simulink model "BlockDiagram"  (R2023a)
settings: Solver=VariableStepAuto  StartTime=0.0  StopTime=10.0  RelTol=1e-3
libraries: visionsinks x3, visionsources x2
settings Model: Creator=thaweesaktrongtirakul  LastModifiedBy=thaweesaktrongtirakul

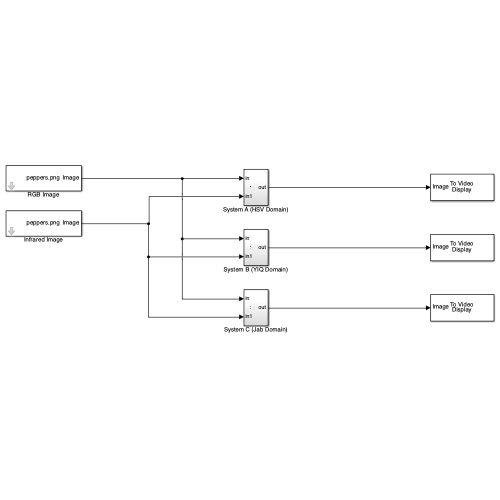
[thumbnail: Simulink's stored preview of the top-level diagram]
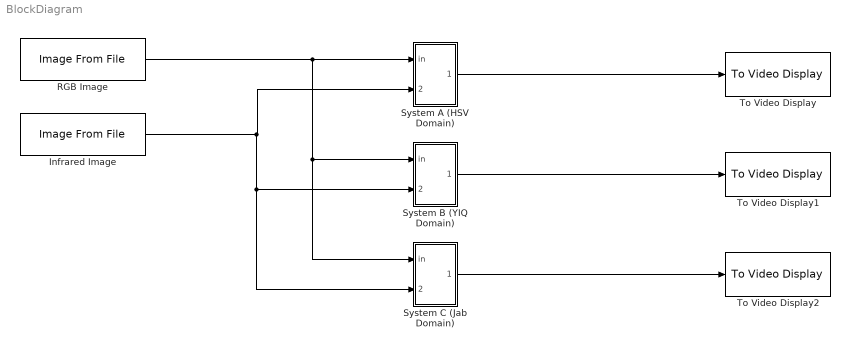
== system BlockDiagram ==
  Infrared Image : visionsources/Image From File  Tag=vipblks_nd  FileName=peppers.png  Ts=inf  imagePorts=One multidimensional signal  OutPortLabels=R|G|B  ImageDataType=Inherit from input image  sdImageDataType=uint(8)  Signed=on  WordLength=16  FractionLengthMode=User-defined  FractionLength=15
  RGB Image : visionsources/Image From File  Tag=vipblks_nd  FileName=peppers.png  Ts=inf  imagePorts=One multidimensional signal  OutPortLabels=R|G|B  ImageDataType=Inherit from input image  sdImageDataType=uint(8)  Signed=on  WordLength=16  FractionLengthMode=User-defined  FractionLength=15
  System A (HSV Domain) : Subsystem
  System B (YIQ Domain) : Subsystem
  System C (Jab Domain) : Subsystem
  To Video Display : visionsinks/To Video Display  windowSizeMode=Normal  openAtMdlStart=on  fullScreen=off  videoWindowX=536805376  videoWindowY=536805376  saveWindowSize=off  videoWindowWidth=2147483647  videoWindowHeight=2147483647  inputColorFormat=RGB  inputType=Obsolete  imagePorts=One multidimensional signal  OutputDevice=On-screen video monitor  dataOrg=Column-major  isWindowOpen=off
  To Video Display1 : visionsinks/To Video Display  windowSizeMode=Normal  openAtMdlStart=on  fullScreen=off  videoWindowX=536805376  videoWindowY=536805376  saveWindowSize=off  videoWindowWidth=2147483647  videoWindowHeight=2147483647  inputColorFormat=RGB  inputType=Obsolete  imagePorts=One multidimensional signal  OutputDevice=On-screen video monitor  dataOrg=Column-major  isWindowOpen=off
  To Video Display2 : visionsinks/To Video Display  windowSizeMode=Normal  openAtMdlStart=on  fullScreen=off  videoWindowX=536805376  videoWindowY=536805376  saveWindowSize=off  videoWindowWidth=2147483647  videoWindowHeight=2147483647  inputColorFormat=RGB  inputType=Obsolete  imagePorts=One multidimensional signal  OutputDevice=On-screen video monitor  dataOrg=Column-major  isWindowOpen=off
  wires:
  RGB Image/1 -> System C (Jab Domain)/1(in), System B (YIQ Domain)/1(in), System A (HSV Domain)/1(in)
  Infrared Image/1 -> System C (Jab Domain)/2(in1), System B (YIQ Domain)/2(in1), System A (HSV Domain)/2(in1)
  System A (HSV Domain)/1(out) -> To Video Display/1
  System B (YIQ Domain)/1(out) -> To Video Display1/1
  System C (Jab Domain)/1(out) -> To Video Display2/1

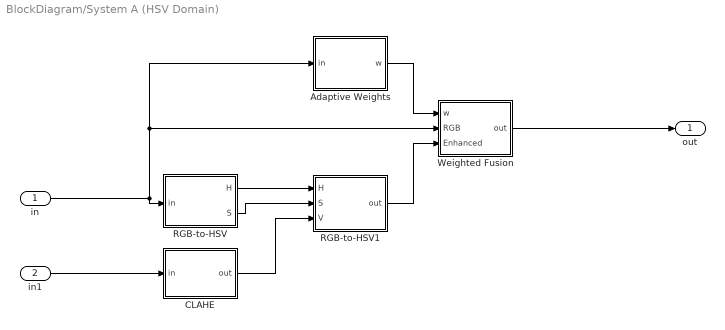
== system BlockDiagram/System A (HSV Domain) ==
  in : Inport
  in1 : Inport  Port=2
  Adaptive Weights : MATLAB Function  TreatAsAtomicUnit=on
  CLAHE : MATLAB Function  TreatAsAtomicUnit=on
  RGB-to-HSV : MATLAB Function  TreatAsAtomicUnit=on
  RGB-to-HSV1 : MATLAB Function  TreatAsAtomicUnit=on
  Weighted Fusion : MATLAB Function  TreatAsAtomicUnit=on
  out : Outport
  wires:
  Weighted Fusion/1(out) -> out/1
  in1/1 -> CLAHE/1(in)
  RGB-to-HSV1/1(out) -> Weighted Fusion/3(Enhanced)
  CLAHE/1(out) -> RGB-to-HSV1/3(V)
  RGB-to-HSV/1(H) -> RGB-to-HSV1/1(H)
  Adaptive Weights/1(w) -> Weighted Fusion/1(w)
  RGB-to-HSV/2(S) -> RGB-to-HSV1/2(S)
  in/1 -> Weighted Fusion/2(RGB), Adaptive Weights/1(in), RGB-to-HSV/1(in)

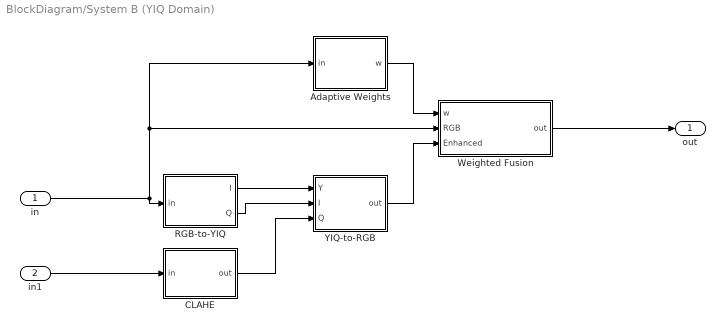
== system BlockDiagram/System B (YIQ Domain) ==
  in : Inport
  in1 : Inport  Port=2
  Adaptive Weights : MATLAB Function  TreatAsAtomicUnit=on
  CLAHE : MATLAB Function  TreatAsAtomicUnit=on
  RGB-to-YIQ : MATLAB Function  TreatAsAtomicUnit=on
  Weighted Fusion : MATLAB Function  TreatAsAtomicUnit=on
  YIQ-to-RGB : MATLAB Function  TreatAsAtomicUnit=on
  out : Outport
  wires:
  Weighted Fusion/1(out) -> out/1
  in1/1 -> CLAHE/1(in)
  YIQ-to-RGB/1(out) -> Weighted Fusion/3(Enhanced)
  CLAHE/1(out) -> YIQ-to-RGB/3(Q)
  RGB-to-YIQ/1(I) -> YIQ-to-RGB/1(Y)
  Adaptive Weights/1(w) -> Weighted Fusion/1(w)
  RGB-to-YIQ/2(Q) -> YIQ-to-RGB/2(I)
  in/1 -> Weighted Fusion/2(RGB), Adaptive Weights/1(in), RGB-to-YIQ/1(in)

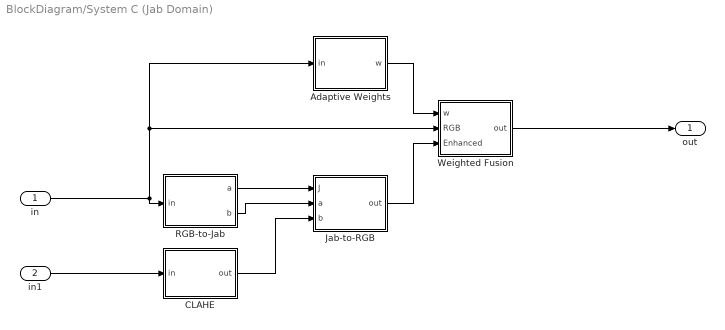
== system BlockDiagram/System C (Jab Domain) ==
  in : Inport
  in1 : Inport  Port=2
  Adaptive Weights : MATLAB Function  TreatAsAtomicUnit=on
  CLAHE : MATLAB Function  TreatAsAtomicUnit=on
  Jab-to-RGB : MATLAB Function  TreatAsAtomicUnit=on
  RGB-to-Jab : MATLAB Function  TreatAsAtomicUnit=on
  Weighted Fusion : MATLAB Function  TreatAsAtomicUnit=on
  out : Outport
  wires:
  Weighted Fusion/1(out) -> out/1
  in1/1 -> CLAHE/1(in)
  Jab-to-RGB/1(out) -> Weighted Fusion/3(Enhanced)
  CLAHE/1(out) -> Jab-to-RGB/3(b)
  RGB-to-Jab/1(a) -> Jab-to-RGB/1(J)
  Adaptive Weights/1(w) -> Weighted Fusion/1(w)
  RGB-to-Jab/2(b) -> Jab-to-RGB/2(a)
  in/1 -> Weighted Fusion/2(RGB), Adaptive Weights/1(in), RGB-to-Jab/1(in)

== matlab function BlockDiagram/System C (Jab Domain)/Weighted Fusion ==
  data: w input; RGB input; out output; Enhanced input
function out = fcn(w,RGB,Enhanced)
    out = RGB+Enhanced+w;
end

== matlab function BlockDiagram/System A (HSV Domain)/RGB-to-HSV ==
  data: in input; H output; S output
function [H,S] = fcn(in)
    H = in;
    S = in;

end

== matlab function BlockDiagram/System C (Jab Domain)/RGB-to-Jab ==
  data: in input; a output; b output
function [a,b] = fcn(in)
    a = in;
    b = in;

end

== matlab function BlockDiagram/System C (Jab Domain)/Jab-to-RGB ==
  data: J input; out output; a input; b input
function out = fcn(J,a,b)
    out = J+a+b;
end

== matlab function BlockDiagram/System A (HSV Domain)/CLAHE ==
  data: in input; out output
function out = fcn(in)
    out = in;
end

== matlab function BlockDiagram/System A (HSV Domain)/RGB-to-HSV1 ==
  data: H input; out output; S input; V input
function out = fcn(H,S,V)
    out = H+S+V;
end

== matlab function BlockDiagram/System A (HSV Domain)/Adaptive Weights ==
  data: in input; w output
function w  = fcn(in)
    w = in;
end

== matlab function BlockDiagram/System A (HSV Domain)/Weighted Fusion ==
  data: w input; RGB input; out output; Enhanced input
function out = fcn(w,RGB,Enhanced)
    out = RGB+Enhanced+w;
end

== matlab function BlockDiagram/System B (YIQ Domain)/Adaptive Weights ==
  data: in input; w output
function w  = fcn(in)
    w = in;
end

== matlab function BlockDiagram/System B (YIQ Domain)/CLAHE ==
  data: in input; out output
function out = fcn(in)
    out = in;
end

== matlab function BlockDiagram/System B (YIQ Domain)/Weighted Fusion ==
  data: w input; RGB input; out output; Enhanced input
function out = fcn(w,RGB,Enhanced)
    out = RGB+Enhanced+w;
end

== matlab function BlockDiagram/System B (YIQ Domain)/RGB-to-YIQ ==
  data: in input; I output; Q output
function [I,Q] = fcn(in)
    I = in;
    Q = in;

end

== matlab function BlockDiagram/System B (YIQ Domain)/YIQ-to-RGB ==
  data: Y input; out output; I input; Q input
function out = fcn(Y,I,Q)
    out = Y+I+Q;
end

== matlab function BlockDiagram/System C (Jab Domain)/Adaptive Weights ==
  data: in input; w output
function w  = fcn(in)
    w = in;
end

== matlab function BlockDiagram/System C (Jab Domain)/CLAHE ==
  data: in input; out output
function out = fcn(in)
    out = in;
end
